simulink model "state_space_simulink_feedforward_control101"  (R2023b)
settings: Solver=VariableStepAuto  StartTime=0.0  StopTime=10.0  RelTol=1e-3
undefined symbols (not defined in the file or in its folder): A, B, C, Cx, Dx, K, P
settings Model: Creator=Anthony  LastModifiedBy=Anthony Rossiter
settings DataIOCC: SaveFormat=StructureWithTime  SignalLogging=off
settings ModelReferenceCC: EnableRefExpFcnMdlSchedulingChecks=on

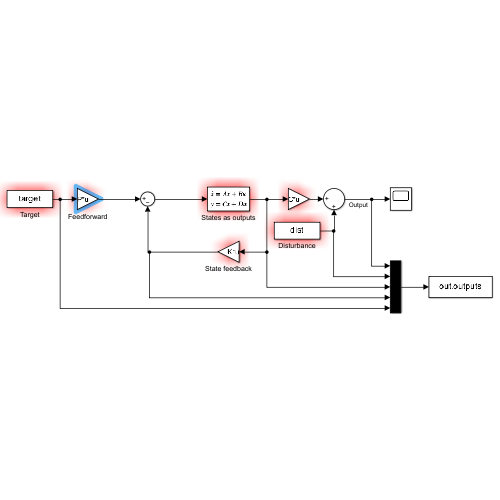
[thumbnail: Simulink's stored preview of the top-level diagram]
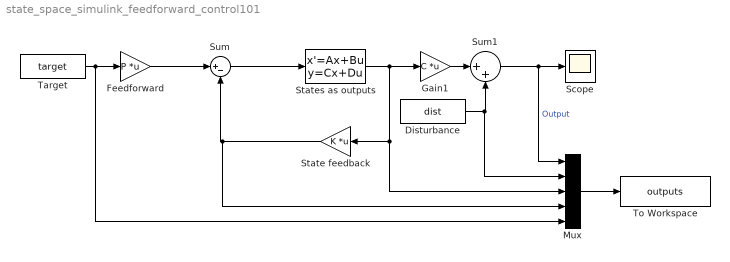
== system state_space_simulink_feedforward_control101 ==
  Disturbance : FromWorkspace  VariableName=dist
  Feedforward : Gain  Gain=P  Multiplication=Matrix(K*u)
  Gain1 : Gain  Gain=C  Multiplication=Matrix(K*u)
  Mux : Mux  Inputs=5
  Scope : Scope
  State feedback : Gain  Gain=K  Multiplication=Matrix(K*u)
  States as outputs : StateSpace  A=A  B=B  C=Cx  D=Dx  InitialCondition=0
  Sum : Sum  Inputs=|+-
  Sum1 : Sum  Inputs=|++
  Target : FromWorkspace  VariableName=target
  To Workspace : ToWorkspace  VariableName=outputs  SaveFormat=Structure With Time  SampleTime=-1
  wires:
  States as outputs/1 -> Gain1/1, Mux/3, State feedback/1
  State feedback/1 -> Mux/4, Sum/2
  Sum/1 -> States as outputs/1
  Feedforward/1 -> Sum/1
  Gain1/1 -> Sum1/1
  Sum1/1 -> Mux/1, Scope/1  "Output"
  Target/1 -> Mux/5, Feedforward/1
  Disturbance/1 -> Mux/2, Sum1/2
  Mux/1 -> To Workspace/1
